simulink model "rlc_test"  (R2019a)
settings: Solver=VariableStepAuto  StartTime=0.0  StopTime=10.0  RelTol=1e-3
libraries: simulink x1
settings Model: Creator=rosha  LastModifiedBy=rosha

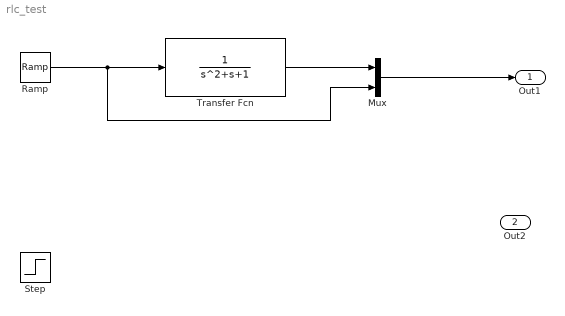
== system rlc_test ==
  Mux : Mux  Inputs=2
  Ramp : simulink/Sources/Ramp  slope=1  start=0  InitialOutput=0
  Step : Step  SampleTime=0
  Transfer Fcn : TransferFcn  Denominator=[1 1 1]
  Out1 : Outport
  Out2 : Outport  Port=2
  wires:
  Ramp/1 -> Transfer Fcn/1, Mux/2
  Transfer Fcn/1 -> Mux/1
  Mux/1 -> Out1/1
